simulink model "ModularStruct"  (R2015a)
settings: Solver=FixedStepDiscrete  StartTime=0.0  StopTime=tsim  FixedStep=dt  RelTol=1e-3
values from neighbouring files (symbols this model uses):
  Cond_bot_T_IC = [(10^-9)*ones(n_bot,1) zeros(n_bot,1)]    [run_ModularStruct.m]
  Cond_top_B_IC = [(10^-9)*ones(n_top,1) zeros(n_top,1)]    [run_ModularStruct.m]
  Conv_bot_B = [Tb_bot*ones(n_bot,1) hb_top*ones(n_bot,1)]    [run_ModularStruct.m]
  Conv_bot_L = [Tl_bot*ones(m_bot,1) hl_bot*ones(m_bot,1)]    [run_ModularStruct.m]
  Conv_bot_R = [Tr_bot*ones(m_bot,1) hr_bot*ones(m_bot,1)]    [run_ModularStruct.m]
  Conv_top_B = [Tb_top*ones(n_top,1) [hb_top*ones(7,1); zeros(8,1); hb_top*ones(7,1)]]    [run_ModularStruct.m]
  Conv_top_L = [Tl_top*ones(m_top,1) hl_top*ones(m_top,1)]    [run_ModularStruct.m]
  Conv_top_R = [Tr_top*ones(m_top,1) hr_top*ones(m_top,1)]    [run_ModularStruct.m]
  Conv_top_T = [Tt_top*ones(n_top,1) ht_top*ones(n_top,1)]    [run_ModularStruct.m]
  Cp2d_bot = Cp*ones(length(y0_bot),length(x_bot))    [run_ModularStruct.m]
  Cp2d_top = Cp*ones(length(y0_top),length(x_top))    [run_ModularStruct.m]
  k2d_bot = k*ones(length(y0_bot),length(x_bot))    [run_ModularStruct.m]
  k2d_top = k*ones(length(y0_top),length(x_top))    [run_ModularStruct.m]
  m_bot = 20    [run_ModularStruct.m]
  rho2d_bot = rho*ones(length(y0_bot),length(x_bot))    [run_ModularStruct.m]
  rho2d_top = rho*ones(length(y0_top),length(x_top))    [run_ModularStruct.m]
undefined symbols (not defined in the file or in its folder): Cind_bot
libraries: lib_Conduction_2DCondFullyImplicit x2
settings Model: Creator=jlkratz  LastModifiedBy=jlkratz

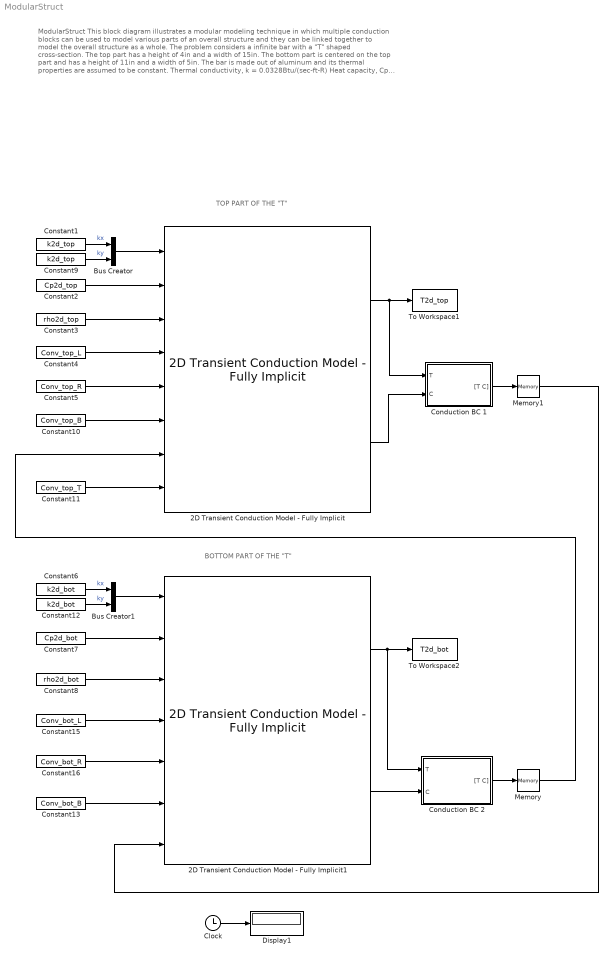
== system ModularStruct ==
  note: TOP PART OF THE "T"
  note: ModularStruct
      |
      | This block diagram illustrates a modular modeling technique in which multiple conduction blocks can be used to
      | model various parts of an overall structure and they can be linked together to model the overall structure as a whole.
      |
      | The problem considers a infinite bar with a "T" shaped cross-section. The top part has a height of 4in and a width
      | of 15in. The bottom part is centered on the top part and has a height of 11in and a width of 5in. The bar is made
      | out of aluminum and its thermal properties are assumed to be constant.
      | Thermal conductivity, k = 0.0328Btu/(sec-ft-R)
      | Heat capacity, Cp = 6.92Btu/(slug-R)
      | Density, rho = 5.24slug/ft^3
      | The plate is at an initial temperature of 550R throughout. It is heated on all sides by convection via a fluid with a
      | temperature of 850R and a heat transfer coefficient of 0.05Btu/(sec-ft^2-R)
  note: BOTTOM PART OF THE "T"
  2D Transient Conduction Model - Fully Implicit : lib_Conduction_2DCondFullyImplicit/2D Transient Conduction Model - Fully Implicit  T0_M=T02d_top  dt_M=dt  x_M=x_top  y_M=y0_top  shape_M=Planar in both directions  convL_M=on  radL_M=off  condL_M=off  convR_M=on  radR_M=off  condR_M=off  convB_M=on  radB_M=off  condB_M=on  convT_M=on  radT_M=off  condT_M=off  BN_M=double(gcb)
  2D Transient Conduction Model - Fully Implicit1 : lib_Conduction_2DCondFullyImplicit/2D Transient Conduction Model - Fully Implicit  T0_M=T02d_bot  dt_M=dt  x_M=x_bot  y_M=y0_bot  shape_M=Planar in both directions  convL_M=on  radL_M=off  condL_M=off  convR_M=on  radR_M=off  condR_M=off  convB_M=on  radB_M=off  condB_M=off  convT_M=off  radT_M=off  condT_M=on  BN_M=double(gcb)
  Bus Creator : BusCreator  Inputs=2
  Bus Creator1 : BusCreator  Inputs=2
  Clock : Clock
  Conduction BC 1 : Subsystem
  Conduction BC 2 : Subsystem
  Constant1 : Constant  Value=k2d_top
  Constant10 : Constant  Value=Conv_top_B
  Constant11 : Constant  Value=Conv_top_T
  Constant12 : Constant  Value=k2d_bot
  Constant13 : Constant  Value=Conv_bot_B
  Constant15 : Constant  Value=Conv_bot_L
  Constant16 : Constant  Value=Conv_bot_R
  Constant2 : Constant  Value=Cp2d_top
  Constant3 : Constant  Value=rho2d_top
  Constant4 : Constant  Value=Conv_top_L
  Constant5 : Constant  Value=Conv_top_R
  Constant6 : Constant  Value=k2d_bot
  Constant7 : Constant  Value=Cp2d_bot
  Constant8 : Constant  Value=rho2d_bot
  Constant9 : Constant  Value=k2d_top
  Display1 : Display
  Memory : Memory  X0=Cond_top_B_IC
  Memory1 : Memory  X0=Cond_bot_T_IC
  To Workspace1 : ToWorkspace  VariableName=T2d_top  SaveFormat=Timeseries  SampleTime=-1
  To Workspace2 : ToWorkspace  VariableName=T2d_bot  SaveFormat=Timeseries  SampleTime=-1
  wires:
  Constant1/1 -> Bus Creator/1  "kx"
  Constant9/1 -> Bus Creator/2  "ky"
  Bus Creator/1 -> 2D Transient Conduction Model - Fully Implicit/1
  Constant2/1 -> 2D Transient Conduction Model - Fully Implicit/2
  Constant3/1 -> 2D Transient Conduction Model - Fully Implicit/3
  Constant11/1 -> 2D Transient Conduction Model - Fully Implicit/8
  Constant10/1 -> 2D Transient Conduction Model - Fully Implicit/6
  2D Transient Conduction Model - Fully Implicit/1 -> Conduction BC 1/1(T), To Workspace1/1
  Constant4/1 -> 2D Transient Conduction Model - Fully Implicit/4
  Constant5/1 -> 2D Transient Conduction Model - Fully Implicit/5
  Clock/1 -> Display1/1
  2D Transient Conduction Model - Fully Implicit1/1 -> Conduction BC 2/1(T), To Workspace2/1
  Constant6/1 -> Bus Creator1/1  "kx"
  Constant12/1 -> Bus Creator1/2  "ky"
  Bus Creator1/1 -> 2D Transient Conduction Model - Fully Implicit1/1
  Constant7/1 -> 2D Transient Conduction Model - Fully Implicit1/2
  Constant8/1 -> 2D Transient Conduction Model - Fully Implicit1/3
  Constant13/1 -> 2D Transient Conduction Model - Fully Implicit1/6
  Constant15/1 -> 2D Transient Conduction Model - Fully Implicit1/4
  Constant16/1 -> 2D Transient Conduction Model - Fully Implicit1/5
  2D Transient Conduction Model - Fully Implicit/2 -> Conduction BC 1/2(C)
  2D Transient Conduction Model - Fully Implicit1/2 -> Conduction BC 2/2(C)
  Conduction BC 2/1("[T C]") -> Memory/1
  Conduction BC 1/1("[T C]") -> Memory1/1
  Memory/1 -> 2D Transient Conduction Model - Fully Implicit/7
  Memory1/1 -> 2D Transient Conduction Model - Fully Implicit1/7

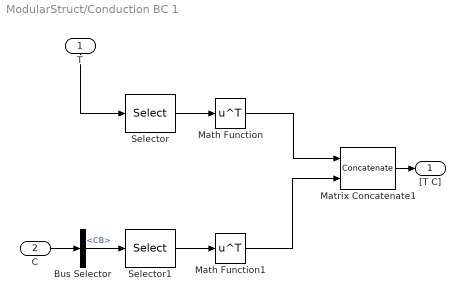
== system ModularStruct/Conduction BC 1 ==
  T : Inport
  C : Inport  Port=2
  Bus Selector : BusSelector  OutputSignals=CB
  Math Function : Math  Operator=transpose  SaturateOnIntegerOverflow=on
  Math Function1 : Math  Operator=transpose  SaturateOnIntegerOverflow=on
  Matrix Concatenate1 : Concatenate  Mode=Multidimensional array  ConcatenateDimension=2
  Selector : Selector  NumberOfDimensions=2  InputPortWidth=3  IndexOptions=Index vector (dialog),Index vector (dialog)  Indices=1,[8:15]  OutputSizes=1,1
  Selector1 : Selector  NumberOfDimensions=2  InputPortWidth=3  IndexOptions=Index vector (dialog),Index vector (dialog)  Indices=1,[8:15]  OutputSizes=1,1
  "[T C]" : Outport
  wires:
  Selector/1 -> Math Function/1
  C/1 -> Bus Selector/1
  Matrix Concatenate1/1 -> "[T C]"/1
  T/1 -> Selector/1
  Bus Selector/1 -> Selector1/1  "<CB>"
  Math Function/1 -> Matrix Concatenate1/1
  Selector1/1 -> Math Function1/1
  Math Function1/1 -> Matrix Concatenate1/2

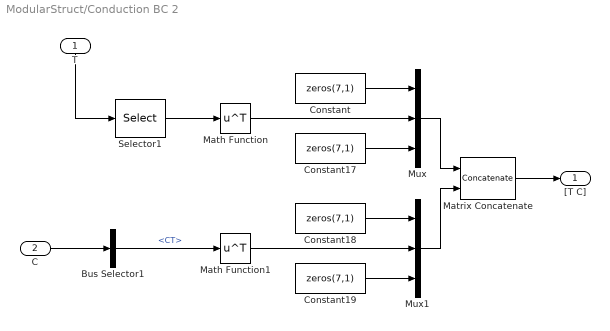
== system ModularStruct/Conduction BC 2 ==
  T : Inport
  C : Inport  Port=2
  Bus Selector1 : BusSelector  OutputSignals=CT
  Constant{,17..19} (4 alike) : Constant  Value=zeros(7,1)
  Math Function : Math  Operator=transpose  SaturateOnIntegerOverflow=on
  Math Function1 : Math  Operator=transpose  SaturateOnIntegerOverflow=on
  Matrix Concatenate : Concatenate  Mode=Multidimensional array  ConcatenateDimension=2
  Mux : Mux  Inputs=3
  Mux1 : Mux  Inputs=3
  Selector1 : Selector  NumberOfDimensions=2  InputPortWidth=3  IndexOptions=Index vector (dialog),Select all  Indices=m_bot,Cind_bot  OutputSizes=1,1
  "[T C]" : Outport
  wires:
  Constant19/1 -> Mux1/3
  Bus Selector1/1 -> Math Function1/1  "<CT>"
  Selector1/1 -> Math Function/1
  Mux/1 -> Matrix Concatenate/1
  Mux1/1 -> Matrix Concatenate/2
  Constant18/1 -> Mux1/1
  Constant/1 -> Mux/1
  Matrix Concatenate/1 -> "[T C]"/1
  Constant17/1 -> Mux/3
  T/1 -> Selector1/1
  C/1 -> Bus Selector1/1
  Math Function/1 -> Mux/2
  Math Function1/1 -> Mux1/2
